simulink model "HingedPendulamControl"  (R2019a)
settings: Solver=FixedStepAuto  StartTime=0.0  StopTime=inf  FixedStep=0.00001  RelTol=1e-3
settings Model: NumberOfSteps=16  Creator=vardhah  LastModifiedBy=vardhah
settings DataIOCC: ReturnWorkspaceOutputs=off
settings DebuggingCC: UnderSpecifiedDimensionMsg=warning  ArithmeticOperatorsInVariantConditions=warning

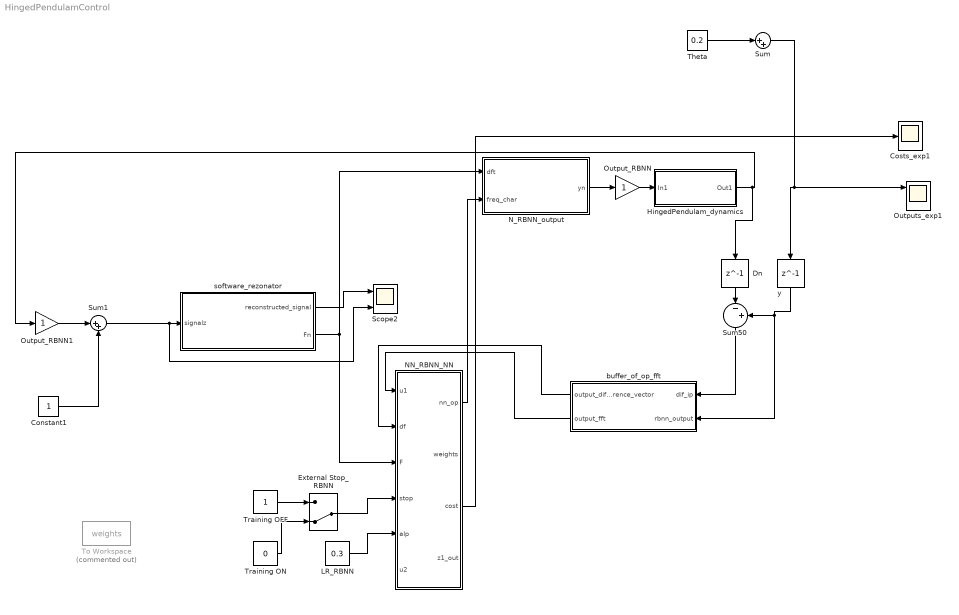
== system HingedPendulamControl ==
  Constant1 : Constant
  Costs_exp1 : Scope
  Dn : Delay  DelayLength=1  InitialCondition=0
  External Stop_RBNN : ManualSwitch  CurrentSetting=0
  HingedPendulam_dynamics : Subsystem
  LR_RBNN : Constant  Value=0.3
  NN_RBNN_NN : MATLAB Function  TreatAsAtomicUnit=on
  N_RBNN_output : MATLAB Function  TreatAsAtomicUnit=on
  Output_RBNN : Gain
  Output_RBNN1 : Gain
  Outputs_exp1 : Scope  NumInputPorts=2
  Scope2 : Scope  NumInputPorts=2
  Sum : Sum  Inputs=|++
  Sum1 : Sum  Inputs=|++
  Sum50 : Sum  Inputs=|-+
  Theta : Constant  Value=0.2
  To Workspace : ToWorkspace  Commented=on  VariableName=weights  SaveFormat=Timeseries  SampleTime=-1
  Training OFF : Constant
  Training ON : Constant  Value=0
  buffer_of_op_fft : MATLAB Function  TreatAsAtomicUnit=on
  software_rezonator : MATLAB Function  TreatAsAtomicUnit=on
  y : Delay  DelayLength=1  InitialCondition=0
  wires:
  software_rezonator/1(reconstructed_signal) -> Scope2/1
  software_rezonator/2(Fn) -> NN_RBNN_NN/3(F), N_RBNN_output/1(dft)
  N_RBNN_output/1(yn) -> Output_RBNN/1
  Dn/1 -> Sum50/1
  y/1 -> Sum50/2, buffer_of_op_fft/2(rbnn_output)
  NN_RBNN_NN/1(nn_op) -> N_RBNN_output/2(freq_char)
  External Stop_RBNN/1 -> NN_RBNN_NN/4(stop)
  Training OFF/1 -> External Stop_RBNN/1
  Training ON/1 -> External Stop_RBNN/2
  NN_RBNN_NN/3(cost) -> Costs_exp1/1
  Sum50/1 -> buffer_of_op_fft/1(dif_ip)
  buffer_of_op_fft/1(output_difference_vector) -> NN_RBNN_NN/2(df)
  LR_RBNN/1 -> NN_RBNN_NN/5(alp)
  buffer_of_op_fft/2(output_fft) -> NN_RBNN_NN/1(u1)
  Sum/1 -> y/1, Outputs_exp1/1
  Sum1/1 -> Scope2/2, software_rezonator/1(signalz)
  Theta/1 -> Sum/1
  Constant1/1 -> Sum1/2
  Output_RBNN/1 -> HingedPendulam_dynamics/1(In1)
  HingedPendulam_dynamics/1(Out1) -> Dn/1, Output_RBNN1/1
  Output_RBNN1/1 -> Sum1/1

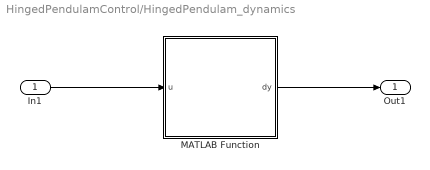
== system HingedPendulamControl/HingedPendulam_dynamics ==
  In1 : Inport
  MATLAB Function : MATLAB Function  TreatAsAtomicUnit=on
  Out1 : Outport
  wires:
  MATLAB Function/1(dy) -> Out1/1
  In1/1 -> MATLAB Function/1(u)

== matlab function HingedPendulamControl/HingedPendulam_dynamics/MATLAB Function ==
  data: u input; dy output
function dy = cartpend(u)
persistent y; 

if isempty(y) 
    y= [0 ; 0 ; 0 ;1];
end


m = 1;
M = 5;
L = 2;
g = -10;
d = 1;

Sy = sin(y(3));
Cy = cos(y(3));
D = m*L*L*(M+m*(1-Cy^2));

dy(1,1) = y(2);
dy(2,1) = (1/D)*(-m^2*L^2*g*Cy*Sy + m*L^2*(m*L*y(4)^2*Sy - d*y(2))) + m*L*L*(1/D)*u;
dy(3,1) = y(4);
dy(4,1) = (1/D)*((m+M)*m*g*L*Sy - m);

== matlab function HingedPendulamControl/NN_RBNN_NN ==
  settings: sampleTime=0.01
  data: u1 input; df input; F input; nn_op output; weights output; cost output; z1_out output; stop input; alp input; u2 input
function [nn_op,weights,cost,z1_out]  = NN(u1,df,F,stop,alp,u2)

persistent w1 w2 w3;
persistent vy;
persistent g1 g2 g3;
persistent itr;
persistent J;
persistent del_w1 del_w2 del_w3;
persistent mult1 mult2 mult3;
persistent memory_alloc_flag;
persistent n;

%%
%%%%%%----------------------------------------------------------------------------%%%%%
%Hyper-parameter & other tunable part of code

M=16;   %declare batch size of training (It will also be equal to number of input in our case as we are using DFT)
%E=16;    % size of external associative input

%layer declaration
layer_1=16;
layer_2=16;
layer_3=16;       % Output layer must match with number of rezonators declared in rezonator function

%learning rate. Currently reading from input pin 
alpha = alp;

%others
input_layer =M;       %layer_0
output_layer=layer_3;

% weight Intialisation 
if isempty(w1)
       w1=randn(input_layer,layer_1)*0.1;
end
if isempty(w2)
       w2=randn(layer_1,layer_2)*0.1;
end
if isempty(w3)
       w3=randn(layer_2,layer_3)*0.1;
end

%%%%%---------------------------------------------------------------------------------%%%%%

%%

%synchronising clock
if isempty(n)
        n = 0; end
n=n+1;

%%
%Allocation of variables that will be used during runtime( one time execution code) 
if isempty(memory_alloc_flag)
        memory_alloc_flag = 0; 
end
if isempty(mult1)
       mult1=zeros(layer_1,layer_1*input_layer); 
end
if isempty(mult2)
       mult2=zeros(layer_2,layer_1*layer_2); 
end
if isempty(mult3)
       mult3=zeros(layer_3,layer_2*layer_3); 
end
if isempty(vy)
       vy=zeros(input_layer,M); 
end

if memory_alloc_flag==0
 %write memory allocation for looped code here.It runs once and store it in memory.  
 mult1=[];
 mult2=[];
 mult3=[];
  for iteration =1:layer_1
   mult1=[mult1;[zeros(1,(iteration-1)*input_layer) ones(1,input_layer) zeros(1,(layer_1-iteration)*input_layer)]];
  end
  for iterate=1:layer_2
   mult2=[mult2;[zeros(1,(iterate-1)*layer_1) ones(1,layer_1) zeros(1,(layer_2-iterate)*layer_1)]];
  end
  for iterate=1:layer_3
   mult3=[mult3;[zeros(1,(iterate-1)*layer_2) ones(1,layer_2) zeros(1,(layer_3-iterate)*layer_2)]];
  end
%{ 
 for k= 1:input_layer
    for j = 1:M 
        if k<=(M/2)+1 && k>=1
            vy(k,j)=(1/M)*cos(pi*(M-j)*(k-1)/(M/2));
        elseif k<=M && k>=(M/2)+1
            vy(k,j)=-(1/M)*sin(pi*(M-j)*(k-1)/(M/2));
        elseif k>M
            vy(k,j)=0;     
        end
    end
 end
 %}
 memory_alloc_flag=1; 
end

%%
%============All other Initiaisation =========================>

%Initialisation of delta of weight storage
if isempty(del_w1)
    del_w1=zeros(1,input_layer*layer_1);
end
if isempty(del_w2)
    del_w2=zeros(1,layer_2*layer_1);
end
if isempty(del_w3)
    del_w3=zeros(1,layer_2*layer_3);
end

%Intialising iteration number & cost value. 
if isempty(itr)
    itr=0;
end
if isempty(J)
    J=0;
end


%gradient initialisation(in matrix form)
if isempty(g1)
    g1= zeros(M,input_layer*layer_1);   
end
if isempty(g2)
    g2= zeros(M,layer_1*layer_2);   
end
if isempty(g3)
    g3= zeros(M,layer_3*layer_2);   
end

%%
%Input vector creation code block
%x_in = [real(u1(1:(size(u1,2)/2)+1)) imag(u1(1:(size(u1,2)/2)-1))];
%v=x_in';
v=u1;
%%
%RBNN core vectorised algorithm implementation 

%--------------->forward propogation ------------>

z1=w1'*v ;
a1=(1./(1+exp(-z1)));
an1=(a1-0.5);
z2=w2'*an1 ;
a2=(1./(1+exp(-z2)));
an2=(a2-0.5);
z3=w3'*an2 ;
a3=(1./(1+exp(-z3)));
an3=(a3-0.5);

%-------------> Backward Propogation -------->

%calculation of Nv:
da3_z3=a3.*(1-a3);
dn_a2=w3'.*repmat(da3_z3,1,layer_2);
da2_z2=a2.*(1-a2);
dn_z2= dn_a2.* repmat(transpose(da2_z2),output_layer,1);
dn_a1=dn_z2*w2';
da1_z1=a1.*(1-a1); 
dn_z1=dn_a1.*repmat(transpose(da1_z1),output_layer,1);
dn_v=dn_z1*w1';   %"This is Nv" 

%calculation of aD, A & B 
aD=transpose(F)*dn_v*vy;
A=[aD;eye(M-1) zeros(M-1,1)];
B=[transpose(F) ; zeros(M-1,size(F,1))]; 

%calculation of Nw(diff of N(v,w) wrt each weights)
dIn_3= da3_z3*transpose(a2);
dn_w3=repmat(dIn_3,1,layer_3).* mult3;

dIn_2= da2_z2*transpose(a1);
da2_w2=repmat(dIn_2,1,layer_2).* mult2;
dn_w2=dn_a2*da2_w2;

dIn_1= da1_z1*transpose(v);
da1_w1= repmat(dIn_1,1,layer_1).*mult1;
dn_w1=dn_a1*da1_w1;

%gradient updation
g3=A*g3+B*dn_w3;
g2=A*g2+B*dn_w2;
g1=A*g1+B*dn_w1;

%Training & updation only once in a batch(batch size=M,n=Overall counter) 
if mod(n,M)==0 && stop==0
%if stop==0
    del_w1 =alpha*df*1*g1/M ;
    del_w2 =alpha*df*1*g2/M ;
    del_w3 =alpha*df*1*g3/M ;
    del_w_reshaped1= reshape(del_w1,[input_layer,layer_1]);
    del_w_reshaped2= reshape(del_w2,[layer_1,layer_2]);
    del_w_reshaped3= reshape(del_w3,[layer_2,layer_3]);
    w1=w1+ del_w_reshaped1;
    w2=w2+ del_w_reshaped2;
    w3=w3+ del_w_reshaped3; 
    itr=itr+1;
    J= sum(df.^2,'all')/(2*M);
end

%For logging & visulisation purpose
cost=J;
weights=w1;
z1_out=z1;
z2_out=z2;

%NN output assignment
nn_op=an3;


end

== matlab function HingedPendulamControl/buffer_of_op_fft ==
  data: output_difference_vector output size=[1,16]; output_fft output size=[1,16]; dif_ip input; rbnn_output input
function [output_difference_vector,output_fft] = difBuffer(dif_ip,rbnn_output)                      

 sz=16;                       % size of the dft 
 
 persistent a;
 persistent b;
 if isempty(b)
  b= zeros(1,sz);
 end
 if isempty(a)
  a= zeros(1,sz);
 end
 
 
  a= circshift(a,1);
  a(1)=dif_ip;
  b= circshift(b,1);
  b(1)=rbnn_output;

 output_difference_vector=a; 
 output_fft=b;
end

== matlab function HingedPendulamControl/software_rezonator ==
  data: signalz input; reconstructed_signal output; Fn output size=16
function [reconstructed_signal,Fn]   = rezonator(signalz)

persistent numberofrezonator;
persistent g c bfr_rezo_sm aft_delay dft_out;
persistent out signal_dif;
persistent n;
persistent memory_alloc_flag;


%assign the number of rezonator here. For configuring it for higher order
%rezonator  we need to change (1) 'numberofrezonaotor' variable
if isempty(numberofrezonator)
        numberofrezonator = 16;   %here 16 parallel rezonators
end
N=16;
%Initialisation of memory allocations/variables ====> 
if isempty(memory_alloc_flag)
        memory_alloc_flag = 0; 
end
if isempty(g)
       g=zeros(numberofrezonator,numberofrezonator,'like',0i); 
end
if isempty(c)
       c=zeros(numberofrezonator,numberofrezonator,'like',0i); 
end
if memory_alloc_flag==0
 for i=0:numberofrezonator-1
  for j= 0:numberofrezonator-1
   g(i+1,j+1)=1/numberofrezonator*(exp(-1i*2*pi*i*j/numberofrezonator));
   c(i+1,j+1)=(exp(1i*2*pi*i*j/numberofrezonator));
  end 
 end
 memory_alloc_flag=1;
end


%Initialisation of variables  =====> 
if isempty(n)
        n = 0;   
end 
if isempty(out)
  out=0+0i;
end
if isempty(signal_dif)
  signal_dif=0+0i;
end
if isempty(bfr_rezo_sm)
  bfr_rezo_sm=repmat(0+0i,numberofrezonator,1);
end
if isempty(aft_delay)
  aft_delay=repmat(0+0i,numberofrezonator,1);
end
if isempty(dft_out)
  dft_out=repmat(0+0i,numberofrezonator,1);
end

%creating cycle of rotation for selection of correct column of g & c.
cycle=mod(n,numberofrezonator);

%resonator core -----------------------------> 
dft_out=c(:,cycle+1).*aft_delay;
out= sum(dft_out,1);
signal_dif=signalz-out;
bfr_rezo_sm=g(:,cycle+1).*signal_dif;

%counting the counter
n=n+1;

% output assignment ------------------>
reconstructed_signal=out;
dft=aft_delay; 
%N=size(dft,1);
a=1:1:N/2-1;
b=N/2+1:1:N-1;
dft_trans=transpose(dft);
Fn=transpose([real(dft_trans(1)) 2*(real(dft_trans(2:N/2)).*cos(2*pi*a*n/N)-imag(dft_trans(2:N/2)).*sin(2*pi*a*n/N)) -1^n*real(dft_trans(N/2+1)) -2*(imag(dft_trans(N/2+2:N)).*cos(2*pi*b*n/N)+real(dft_trans(N/2+2:N)).*sin(2*pi*b*n/N))]);
%--------output assignment over----------<

%final updation of buffer ------>>>>>>>>>>>>
aft_delay= aft_delay+bfr_rezo_sm; 
end

== matlab function HingedPendulamControl/N_RBNN_output ==
  data: dft input; yn output; freq_char input
function yn = fcn(dft,freq_char)
yn=transpose(freq_char)*dft;
end
